simulink model "myo_sfun_one_myo_imu_visualization"  (R2013a)
settings: Solver=ode1  StartTime=0.0  StopTime=inf  FixedStep=0.02  RelTol=1e-3
libraries: myo_lib x2, vrlib x2, rtwinlib x1
settings Model: Creator=Mark Tomaszewski  LastModifiedBy=marktoma
settings OptimizationCC: InlineParams=on
settings GRTTargetCC: ExtMode=on

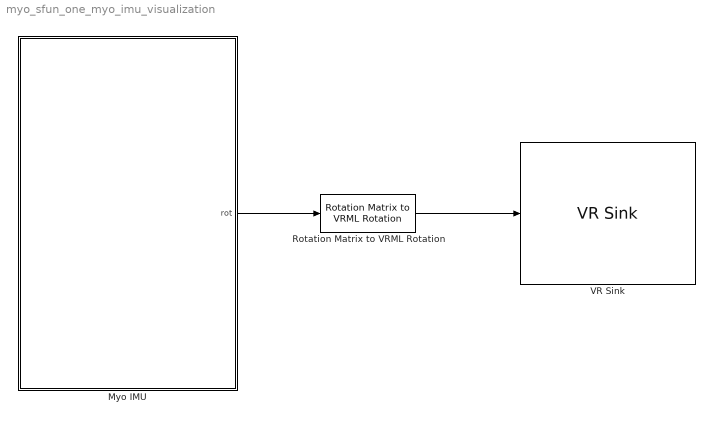
== system myo_sfun_one_myo_imu_visualization ==
  Myo IMU : Subsystem
  Rotation Matrix to VRML Rotation : vrlib/Utilities/Rotation Matrix to VRML Rotation  maxzero=1e-12
  VR Sink : vrlib/VR Sink  InstantiateOnLoad=on  SampleTime=-1  ViewEnable=on  RemoteChange=off  RemoteView=off  FieldsWritten=Myo.rotation.4.1.1.double  WorldFileName=myo_sfun_one_myo_imu_visualization.wrl  AutoView=off  VideoDimensions=[]  AllowVariableSize=off
  wires:
  Myo IMU/1(rot) -> Rotation Matrix to VRML Rotation/1
  Rotation Matrix to VRML Rotation/1 -> VR Sink/1

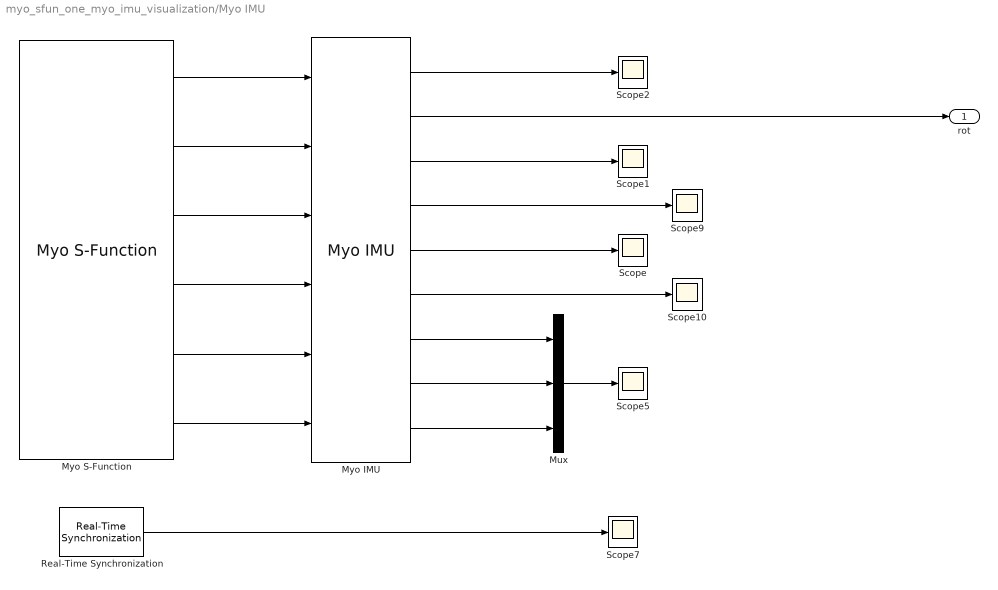
== system myo_sfun_one_myo_imu_visualization/Myo IMU ==
  Mux : Mux  Inputs=3
  Myo IMU : myo_lib/Myo IMU
  Myo S-Function : myo_lib/Myo S-Function  emgEnabled=0  countMyos=1
  Real-Time Synchronization : rtwinlib/Real-Time Synchronization  SampleTime=0.04  MaxMissedTicks=50  ShowMissedTicks=on  YieldWhenWaiting=on
  Scope{,1..2,5,7,9..10} (7 alike) : Scope
      Scope1 settings: YMin=-750  YMax=1750
      Scope10 settings: SaveName=ScopeData10
      Scope2 settings: YMin=-0.4  YMax=0.9  SaveName=ScopeData2
      Scope5 settings: SaveName=ScopeData5
      Scope7 settings: TimeRange=10  YMin=-150  YMax=150  SaveName=ScopeData7
      Scope9 settings: YMin=-1750  YMax=1000  SaveName=ScopeData9
  rot : Outport
  wires:
  Real-Time Synchronization/1 -> Scope7/1
  Myo S-Function/4 -> Myo IMU/4
  Myo IMU/3 -> Scope1/1
  Myo S-Function/1 -> Myo IMU/1
  Myo IMU/6 -> Scope10/1
  Myo IMU/7 -> Mux/1
  Myo IMU/8 -> Mux/2
  Myo IMU/2 -> rot/1
  Myo IMU/9 -> Mux/3
  Myo S-Function/3 -> Myo IMU/3
  Myo S-Function/5 -> Myo IMU/5
  Myo S-Function/2 -> Myo IMU/2
  Myo IMU/5 -> Scope/1
  Mux/1 -> Scope5/1
  Myo IMU/1 -> Scope2/1
  Myo IMU/4 -> Scope9/1
  Myo S-Function/6 -> Myo IMU/6
